simulink model "QPTest5"  (R2021a)
settings: Solver=ode45  StartTime=0.0  StopTime=20  FixedStep=Control_timestep  RelTol=1e-3  AbsTol=1e-6
undefined symbols (not defined in the file): Matlab_version, NXMotion, NXMotion_controltimestep, NXMotion_model, NXMotion_model_n, NXMotion_n, NXMotion_solution, NXMotion_solution_n, Plant_inputs_num, Plant_outputs_num
libraries: simulink x1
(part 2 of 3)

== matlab function QPTest5/MATLAB Function5 ==
  data: A input; B input; Theta0 input; XB input; P0 input; dh input; g output; q input; J input
function g = Performance_Gradient(A, B, Theta0, XB, P0, dh, q, J)
% 优化指标：
%   1) 世界坐标系 z 方向的 Directional Force Manipulability
%   2) 世界坐标系 x-y 平面的 Velocity Transmission
%   3) 世界坐标系 rx-ry 平面的 Rotational Stiffness
%
% q 顺序：
%   q(1:6)   = Stewart 六个电缸长度，单位 mm
%   q(7:13)  = 机械臂七个关节角，单位 deg

    %% -------------------------------------------------
    % 0. 固定输出尺寸与输入整理
    % --------------------------------------------------
    g = zeros(13,1);
    
    mu_const = 0;    %  w_m  10   w_s   3e-4     w_v   0.15
    
    q      = reshape(q,      13, 1);
    J      = reshape(J,       6, 13); 
    A      = reshape(A,       6, 3);
    B      = reshape(B,       6, 3);
    XB     = reshape(XB,      3, 1);
    P0     = reshape(P0,      3, 1);
    dh     = reshape(dh,      7, 4);
    Theta0 = reshape(Theta0,  7, 1);

    %% -------------------------------------------------
    % 1. 调参量
    % --------------------------------------------------
    dt = 1.0e-3;   

    % z 方向 Directional Force Manipulability 权重
    w_m = 1;  

    % rx-ry 方向 Rotational Stiffness 权重
    w_s = 0;  

    % x-y 方向 Velocity Transmission 权重
    w_v = 0; 

    % 离散加速度层缩放：
    %   q_{k+1} ≈ q_k + qdot_k*dt + 0.5*qddot_k*dt^2
    mu = mu_const * 0.5 * dt * dt;

    %% -------------------------------------------------
    % 2. 执行器力/力矩归一化矩阵 S_tau
    % --------------------------------------------------
    F_lim_cyl = 0.7 * [
        30;
        30;
        30;
        30;
        30;
        30
    ];  % N

    tau_lim_arm_Nm = 0.7 * [
        87;
        87;
        87;
        87;
        12;
        12;
        12
    ];  % Nm

    tau_lim_arm = tau_lim_arm_Nm * 1000.0;  % N*mm

    tau_lim = [
        F_lim_cyl;
        tau_lim_arm
    ];

    inv_tau = zeros(13,1);

    for i = 1:13
        inv_tau(i) = 1.0 / max(tau_lim(i), 1.0e-9);
    end

    inv_tau(13) = 0.0;

    S_tau = diag(inv_tau .* inv_tau);

    %% -------------------------------------------------
    % 2.1 关节刚度矩阵 Kq 的逆矩阵 Kq_inv
    % --------------------------------------------------
    k_cyl = 1.0e4 * [
        1;
        1;
        1;
        1;
        1;
        1
    ];  % N/mm

    k_arm_Nm_per_rad = 1.0e3 * [
        1;
        1;
        1;
        1;
        1;
        1;
        1
    ];  % Nm/rad

    k_arm = k_arm_Nm_per_rad * 1000.0;  % N*mm/rad

    k_joint = [
        k_cyl;
        k_arm
    ];

    inv_kq = zeros(13,1);

    for i = 1:13
        inv_kq(i) = 1.0 / max(k_joint(i), 1.0e-9);
    end

    inv_kq(13) = 0.0;

    Kq_inv = diag(inv_kq);

    %% -------------------------------------------------
    % 2.2 关节速度能力矩阵 S_qdot
    % --------------------------------------------------
    ldot_lim = 30.0;       % mm/s
    qdot_arm_lim = 0.50;   % rad/s

    qdot_lim = [
        ldot_lim * ones(6,1);
        qdot_arm_lim * ones(7,1)
    ];

    qdot_lim(13) = 0.0;

    S_qdot = diag(qdot_lim .* qdot_lim);

    h = zeros(13,1);

    h(1:6)  = 1.0e-2;  % Stewart 电缸，单位 mm
    h(7:12) = 1.0e-3;  % 机械臂关节，单位 deg
    h(13)   = 0.0;     % 第 7 关节固定

    qdot0 = zeros(13,1);

    grad_eta_m = zeros(13,1);
    grad_eta_s = zeros(13,1);
    grad_eta_v = zeros(13,1);

    for i = 1:12

        qp = q;
        qm = q;

        qp(i) = qp(i) + h(i);
        qm(i) = qm(i) - h(i);

        qp(13) = Theta0(7);
        qm(13) = Theta0(7);

        [Jp, ~] = System_Kinematics(A, B, XB, P0, dh, Theta0, qp, qdot0);
        [Jm, ~] = System_Kinematics(A, B, XB, P0, dh, Theta0, qm, qdot0);

        % 1) z 方向 Directional Force Manipulability
        eta_m_p = eta_dfm_z_from_J(Jp, S_tau);
        eta_m_m = eta_dfm_z_from_J(Jm, S_tau);

        % 2) rx-ry 方向 Directional Rotational Stiffness
        eta_s_p = eta_stiffness_rxy_from_J(Jp, Kq_inv);
        eta_s_m = eta_stiffness_rxy_from_J(Jm, Kq_inv);

        % 3) x-y 方向 Directional Velocity Transmission
        eta_v_p = eta_velocity_xy_from_J(Jp, S_qdot);
        eta_v_m = eta_velocity_xy_from_J(Jm, S_qdot);

        grad_eta_m(i) = (eta_m_p - eta_m_m) / (2.0 * h(i));
        grad_eta_s(i) = (eta_s_p - eta_s_m) / (2.0 * h(i));
        grad_eta_v(i) = (eta_v_p - eta_v_m) / (2.0 * h(i));
    end

    % 第 7 机械臂关节固定
    grad_eta_m(13) = 0.0;
    grad_eta_s(13) = 0.0;
    grad_eta_v(13) = 0.0;

    %% -------------------------------------------------
    % 5. 输出 QP 线性性能项
    %
    %   g = mu * (w_m * grad_eta_m
    %           + w_s * grad_eta_s
    %           + w_v * grad_eta_v)
    %
    % 其中：
    %   grad_eta_m = ∇q eta_m,z
    %   grad_eta_s = ∇q eta_s,rxy
    %   grad_eta_v = ∇q eta_v,xy
    % --------------------------------------------------
    g = mu * ( ...
          w_m * grad_eta_m ...
        + w_s * grad_eta_s ...
        + w_v * grad_eta_v );

    a=w_m * grad_eta_m';
    b=w_s * grad_eta_s';
    c=w_v * grad_eta_v';

    g(13) = 0.0;

    
end


function eta = eta_stiffness_rxy_from_J(J_ext, Kq_inv)

    J_ext  = reshape(J_ext,   6, 13);
    Kq_inv = reshape(Kq_inv, 13, 13);

    deg2rad = pi / 180.0;
    rad2deg = 180.0 / pi;


    Jk = J_ext;

    % 输出角速度/角位移单位：deg -> rad
    Jk(4:6,:) = Jk(4:6,:) * deg2rad;

    % 机械臂输入关节单位：deg -> rad
    Jk(:,7:13) = Jk(:,7:13) * rad2deg;

    % 第 7 机械臂关节固定
    Jk(:,13) = 0.0;

    Cx = Jk * Kq_inv * Jk.';
    Cx = 0.5 * (Cx + Cx.');

    scale_C = 0.0;
    for r = 1:6
        for c = 1:6
            scale_C = scale_C + Cx(r,c) * Cx(r,c);
        end
    end
    scale_C = sqrt(scale_C);

    reg = 1.0e-10 * max(scale_C, 1.0);

    Kx = (Cx + reg * eye(6)) \ eye(6);
    Kx = 0.5 * (Kx + Kx.');

    KR = Kx(4:6,4:6);
    KR = 0.5 * (KR + KR.');

    KRxy = KR(1:2,1:2);
    KRxy = 0.5 * (KRxy + KRxy.');

    eta = min_eig_sym_2x2(KRxy);

    eta = real(eta);
    eta = max(eta, 1.0e-12);

end



function eta = eta_velocity_xy_from_J(J_ext, S_qdot)


    J_ext  = reshape(J_ext,   6, 13);
    S_qdot = reshape(S_qdot, 13, 13);

    rad2deg = 180.0 / pi;


    Jv = J_ext(1:3,:);


    Jv(:,7:13) = Jv(:,7:13) * rad2deg;


    Jv(:,13) = 0.0;

    Jxy = Jv(1:2,:);

    Mv = Jxy * S_qdot * Jxy.';
    Mv = 0.5 * (Mv + Mv.');

    lambda_min = min_eig_sym_2x2(Mv);
    lambda_min = max(real(lambda_min), 1.0e-12);

    eta = sqrt(lambda_min);

end


function eta = eta_dfm_z_from_J(J_ext, S_tau)

    rad2deg = 180.0 / pi;

    ez = [
        0.0;
        0.0;
        1.0
    ];

    ez = ez / max(norm(ez), 1.0e-12);

    %% -------------------------------------------------
    % 1. 取平动 Jacobian
    % --------------------------------------------------
    Jv = J_ext(1:3,:);

    %% -------------------------------------------------
    % 2. 单位转换
    % --------------------------------------------------
    Jv(:,7:13) = Jv(:,7:13) * rad2deg;

    Jv(:,13) = 0.0;

    %% -------------------------------------------------
    % 3. z 方向 Directional Force Manipulability
    % --------------------------------------------------
    alpha = ez.' * (Jv * S_tau * Jv.') * ez;

    alpha = max(alpha, 1.0e-12);

    eta = 1.0 / sqrt(alpha);

end


function lambda_min = min_eig_sym_2x2(M)

    M = reshape(M, 2, 2);
    M = 0.5 * (M + M.');

    a = M(1,1);
    b = M(1,2);
    c = M(2,2);

    tr_half = 0.5 * (a + c);
    disc = sqrt(0.25 * (a - c) * (a - c) + b * b);

    lambda_min = tr_half - disc;

end



function [J, Jdot_qdot] = System_Kinematics (A, B, XB, P0, dh, Theta0, q, qdot)


    %% 0. 输入整理
    J = zeros(6,13);
    Jdot_qdot = zeros(6,1);

    A      = reshape(A,       6, 3);
    B      = reshape(B,       6, 3);
    XB     = reshape(XB,      3, 1);
    P0     = reshape(P0,      3, 1);
    dh     = reshape(dh,      7, 4);
    Theta0 = reshape(Theta0,  7, 1);
    q      = reshape(q,      13, 1);
    qdot   = reshape(qdot,   13, 1);

    deg2rad = pi / 180.0;
    rad2deg = 180.0 / pi;

    %% 1. 构造 qdot13，并强制第 7 机械臂关节速度为 0
    qdot13 = qdot;
    qdot13(13) = 0.0;

    %% 2. 拆分 q 与 qdot
    l_para = q(1:6);             % mm
    q_arm_deg = q(7:13);         % deg

    ldot = qdot13(1:6);          % mm/s
    qdot_arm_deg = qdot13(7:13); % deg/s

    theta7_fixed = Theta0(7);

    q_arm_deg(7) = theta7_fixed;
    qdot_arm_deg(7) = 0.0;

    q_arm_rad = q_arm_deg * deg2rad;
    qdot_arm_rad = qdot_arm_deg * deg2rad;

    %% 3. 几何参数与坐标转换
    A_G0 = A.';             % 3x6
    B_G  = B.';             % 3x6

    XB_G0 = XB(:);          % 3x1
    P0_G  = P0(:);          % 3x1

    A_P = zeros(3,6);
    for i = 1:6
        A_P(:,i) = A_G0(:,i) - P0_G;
    end

    % 机械臂基座 B 相对上平台中心 P 的安装偏置，表达在 {P}
    PpB = XB_G0 - P0_G;     % mm

    PRB = [
        -1.0,  0.0,  0.0;
         0.0, -1.0,  0.0;
         0.0,  0.0,  1.0
    ];

    % dh 中角度列 deg -> rad，长度列保持 mm
    dh_rad = dh;
    dh_rad(:,3) = dh(:,3) * deg2rad;
    dh_rad(:,4) = dh(:,4) * deg2rad;

    %% 4. Stewart 正运动学：由六个电缸长度求当前上平台位姿
    pose_guess_p = P0_G;
    pose_guess_R = eye(3);

    maxIter = 60;
    tol = 1.0e-7;

    [p_GP, R_GP] = stewart_fk_LM( ...
        A_P, B_G, l_para, ...
        pose_guess_p, pose_guess_R, ...
        maxIter, tol);

    %% 5. Stewart 速度雅可比
    [Gq, ~, ~, ~] = stewart_Gq(A_P, B_G, p_GP, R_GP);

    lambda_dls = 1.0e-3;
    A_dls  = Gq.' * Gq + lambda_dls^2 * eye(6);
    J_para = A_dls \ Gq.';

    %% 6. 机械臂 Jacobian，表达在机械臂基坐标系 {B}
    % --------------------------------------------------

    X_AEnd0_G = [-1161.7884; 0.0001; 1560.2205];

    q_arm0_deg = Theta0(:);
    q_arm0_deg(7) = Theta0(7);
    q_arm0_rad = q_arm0_deg * deg2rad;

    % 初始 MDH 末端坐标系 {F} 的位姿，p_tool_F = 0 表示先取 MDH 末端原点
    [~, T_BF0, f_F0_B, ~] = franka_jacobian_mdh_tool( ...
        q_arm0_rad, dh_rad, zeros(3,1));

    R_BF0 = T_BF0(1:3,1:3);

    % 初始时：
    %   X_AEnd0_G = XB_G0 + PRB * (f_F0_B + R_BF0*p_AEnd_F)
    %
    % 因此：
    %   p_AEnd_F = R_BF0' * ( PRB'*(X_AEnd0_G-XB_G0) - f_F0_B )
    p_AEnd_F = R_BF0.' * (PRB.' * (X_AEnd0_G - XB_G0) - f_F0_B);

    % 当前真实控制点 AEnd 的机械臂雅可比
    [J_arm_B_full, ~, f_B, Tlist] = franka_jacobian_mdh_tool( ...
        q_arm_rad, dh_rad, p_AEnd_F);
 
    % 第 7 关节固定：保留其位姿影响，但去掉速度列
    J_arm_B = J_arm_B_full;
    J_arm_B(:,7) = 0.0;

    %% 7. 组合系统总 Jacobian，内部先用 [mm/s; rad/s]
    % ^G R_B = ^G R_P * ^P R_B
    R_B = R_GP * PRB;

    % 从 P 到 AEnd 的向量，表达在 {G}
    r_PF = R_GP * PpB + R_B * f_B;

    G_PF = zeros(6,6);
    G_PF(1:3,1:3) = eye(3);
    G_PF(1:3,4:6) = -skew3(r_PF);
    G_PF(4:6,4:6) = eye(3);

    Rbar_B = zeros(6,6);
    Rbar_B(1:3,1:3) = R_B;
    Rbar_B(4:6,4:6) = R_B;

    J_stew_internal = G_PF  * J_para;
    J_arm_internal  = Rbar_B * J_arm_B;
    J_internal = [J_stew_internal, J_arm_internal];

    D_in = diag([ ...
        1; 1; 1; 1; 1; 1; ...
        deg2rad; deg2rad; deg2rad; deg2rad; deg2rad; deg2rad; deg2rad]);

    D_out = diag([1; 1; 1; rad2deg; rad2deg; rad2deg]);

    J = D_out * J_internal * D_in;
    J(:,13) = 0.0;

    %% 8. 计算 dot(J)*qdot
    % 8.1 Stewart 平台速度
    Xdot_P = J_para * ldot;
    v_P = Xdot_P(1:3);
    w_P = Xdot_P(4:6);

    % 8.2 Stewart 平台 bias 加速度
    dGq_dt  = stewart_dGq_twist(A_P, B_G, p_GP, R_GP, v_P, w_P);
    dJ_para = dls_inverse_dJ(Gq, dGq_dt, lambda_dls, A_dls, J_para);

    Xddot_P = dJ_para * ldot;
    dotv_P = Xddot_P(1:3);
    dotw_P = Xddot_P(4:6);

    % 8.3 机械臂相对 twist 和相对 bias 加速度，表达在 {B}
    Xdot_rel_B = J_arm_B * qdot_arm_rad;
    v_rel_B = Xdot_rel_B(1:3);
    w_rel_B = Xdot_rel_B(4:6);

    Xddot_rel_B = armJdotQdot_geometric_fromTlist_tool( ...
        J_arm_B, Tlist, qdot_arm_rad, f_B);

    dotv_rel_B = Xddot_rel_B(1:3);
    dotw_rel_B = Xddot_rel_B(4:6);

    % 8.4 转到世界坐标系 {G}
    v_rel_G    = R_B * v_rel_B;
    w_rel_G    = R_B * w_rel_B;
    dotv_rel_G = R_B * dotv_rel_B;
    dotw_rel_G = R_B * dotw_rel_B;

    % 8.5 末端 bias 加速度
    dotw_F_internal = dotw_P ...
                    + cross(w_P, w_rel_G) ...
                    + dotw_rel_G;

    dotv_F_internal = dotv_P ...
                    + cross(dotw_P, r_PF) ...
                    + cross(w_P, cross(w_P, r_PF)) ...
                    + 2.0 * cross(w_P, v_rel_G) ...
                    + dotv_rel_G;

    Jdot_qdot_internal = [dotv_F_internal; dotw_F_internal];
    Jdot_qdot = D_out * Jdot_qdot_internal;

    J(:,13) = 0.0;

    
    
    
    
end



%% ========================================================================
%                          Stewart FK: Levenberg-Marquardt
% ========================================================================
function [p, R] = stewart_fk_LM(A_P, B_G, l, p0, R0, maxIter, tol)
% Stewart forward kinematics by LM.
% A_P, B_G, l, p 均为 mm；旋转增量为 rad。

    p = p0(:);
    R = R0;

    lambda = 1.0e-4;
    resPrev = inf;

    for it = 1:maxIter 
        [g, Gq] = stewart_residual_and_Gq(A_P, B_G, p, R, l);
        res = norm(g);

        if res < tol
            break;
        end

        H = Gq.' * Gq + lambda * eye(6);
        delta = -(H \ (Gq.' * g));

        accepted = false;
        for trial = 1:10 
            p_new = p + delta(1:3);
            % 左扰动：delta_phi 为空间角速度/旋转增量，对应 Gq 中 -[R*A]x 项。
            R_new = so3_exp(delta(4:6)) * R;

            g_new = stewart_residual_only(A_P, B_G, p_new, R_new, l);
            res_new = norm(g_new);

            if res_new < res
                p = p_new;
                R = R_new;
                lambda = max(lambda / 5.0, 1.0e-12);
                accepted = true;
                break;
            else
                lambda = lambda * 5.0;
                H = Gq.' * Gq + lambda * eye(6);
                delta = -(H \ (Gq.' * g));
            end
        end

        if ~accepted
            break;
        end

        if abs(resPrev - res) / max(1.0, res) < 1.0e-12
            break;
        end
        resPrev = res;
    end
end

function g = stewart_residual_only(A_P, B_G, p, R, l)
    p = p(:);
    g = zeros(6,1);
    for i = 1:6
        s_i = R * A_P(:,i) + p - B_G(:,i);
        g(i) = norm(s_i) - l(i);
    end
end

function [g, Gq] = stewart_residual_and_Gq(A_P, B_G, p, R, l)
    p = p(:);
    g = zeros(6,1);
    Gq = zeros(6,6);

    rA_G = R * A_P;
    for i = 1:6
        s_i = rA_G(:,i) + p - B_G(:,i);
        L_i = norm(s_i);
        L_i_safe = max(L_i, 1.0e-12);
        u_i = s_i / L_i_safe;

        g(i) = L_i - l(i);
        Gq(i,1:3) = u_i.';
        Gq(i,4:6) = u_i.' * (-skew3(rA_G(:,i)));
    end
end

%% ========================================================================
%                          Stewart velocity Jacobian
% ========================================================================
function [Gq, u_all, rA_G_all, legVec_all] = stewart_Gq(A_P, B_G, p, R)
    p = p(:);

    Gq = zeros(6,6);
    u_all = zeros(3,6);
    rA_G_all = R * A_P;
    legVec_all = zeros(3,6);

    for i = 1:6
        s_i = rA_G_all(:,i) + p - B_G(:,i);
        L_i = norm(s_i);
        L_i_safe = max(L_i, 1.0e-12);
        u_i = s_i / L_i_safe;

        legVec_all(:,i) = s_i;
        u_all(:,i) = u_i;

        Gq(i,1:3) = u_i.';
        Gq(i,4:6) = u_i.' * (-skew3(rA_G_all(:,i)));
    end
end

%% ========================================================================
%                          Franka / 机械臂 MDH Jacobian
% ========================================================================
function [J, T_BF, f_B, Tlist] = franka_jacobian_mdh_tool(q_rad, dh_rad, p_tool_F)

    q_rad = q_rad(:);
    p_tool_F = reshape(p_tool_F, 3, 1);

    theta = q_rad + dh_rad(:,4);

    T = eye(4);
    Tlist = zeros(4,4,7);

    for i = 1:7
        a     = dh_rad(i,1);
        d     = dh_rad(i,2);
        alpha = dh_rad(i,3);
        th    = theta(i);

        Ti = mdh_T(a, d, alpha, th);
        T = T * Ti;
        Tlist(:,:,i) = T;
    end

    T_BF = T;

    R_BF = T_BF(1:3,1:3);
    p_F_B = T_BF(1:3,4);

    % AEnd 点在机械臂基坐标系 {B} 下的位置
    f_B = p_F_B + R_BF * p_tool_F;

    J = zeros(6,7);
    p_e = f_B;

    for i = 1:7
        Ti = Tlist(:,:,i);
        zi = Ti(1:3,3);
        pi = Ti(1:3,4);

        J(1:3,i) = cross(zi, p_e - pi);
        J(4:6,i) = zi;
    end
end

function T = mdh_T(a, d, alpha, theta)
% MDH: Tx(a) * Rx(alpha) * Tz(d) * Rz(theta)
% a,d: mm; alpha,theta: rad
    ca = cos(alpha);
    sa = sin(alpha);
    ct = cos(theta);
    st = sin(theta);

    T = [
        ct,    -st,     0,   a;
        st*ca, ct*ca,  -sa, -d*sa;
        st*sa, ct*sa,   ca,  d*ca;
        0,      0,      0,   1
    ];
end

%% ========================================================================
%                          dot(J_arm)*qdot_arm
% ========================================================================
function Jdotq = armJdotQdot_geometric_fromTlist_tool(J_arm_B, Tlist, qdot_rad, p_e)
% 解析计算机械臂相对项：^B(dot(J_arm)*qdot_arm)
%
% p_e:
%   AEnd 点在机械臂基坐标系 {B} 下的位置，单位 mm。
%
% 输出：
%   前3维 mm/s^2
%   后3维 rad/s^2

    qdot_rad = qdot_rad(:);
    p_e = reshape(p_e, 3, 1);

    n = 7;

    z = zeros(3,n);
    p = zeros(3,n);

    for i = 1:n
        Ti = Tlist(:,:,i);
        z(:,i) = Ti(1:3,3);
        p(:,i) = Ti(1:3,4);
    end

    v_e = J_arm_B(1:3,:) * qdot_rad;

    omega_i = zeros(3,n);
    v_i     = zeros(3,n);

    for i = 1:n
        omega_i(:,i) = z(:,1:i) * qdot_rad(1:i);

        vi = zeros(3,1);
        for k = 1:i
            vi = vi + cross(z(:,k), p(:,i) - p(:,k)) * qdot_rad(k);
        end
        v_i(:,i) = vi;
    end

    vdot_bias = zeros(3,1);
    wdot_bias = zeros(3,1);

    for i = 1:n
        zi = z(:,i);
        pi = p(:,i);

        z_dot = cross(omega_i(:,i), zi);
        wdot_bias = wdot_bias + z_dot * qdot_rad(i);

        vdot_bias = vdot_bias + ...
            ( cross(z_dot, p_e - pi) ...
            + cross(zi, v_e - v_i(:,i)) ) * qdot_rad(i);
    end

    Jdotq = [vdot_bias; wdot_bias];
end

%% ========================================================================
%                          Stewart dGq/dt
% ========================================================================
function dGq = stewart_dGq_twist(A_P, B_G, p, R, v, w)
% 计算 Stewart Gq 的时间导数。
% A_P, B_G, p: mm；v: mm/s；w: rad/s。
% Gq 定义：ldot_i = u_i^T v_P + u_i^T(-[rAi]x) w_P。

    p = p(:);
    v = v(:);
    w = w(:);

    dGq = zeros(6,6);
    rA = R * A_P;

    for i = 1:6
        rAi = rA(:,i);
        s_i = rAi + p - B_G(:,i);

        L_i = norm(s_i);
        L_i_safe = max(L_i, 1.0e-12);
        u_i = s_i / L_i_safe;

        ds = v + cross(w, rAi);
        dL = u_i.' * ds;
        du = (ds - u_i * dL) / L_i_safe;

        drAi = cross(w, rAi);

        dGq(i,1:3) = du.';
        dGq(i,4:6) = du.' * (-skew3(rAi)) ...
                   + u_i.' * (-skew3(drAi));
    end
end

%% ========================================================================
%                          DLS inverse derivative
% ========================================================================
function dJ = dls_inverse_dJ(G, dG, lambda_dls, A, J)
% J = inv(G^T G + lambda^2 I)*G^T 的时间导数。
% dJ = A^{-1} dG^T - A^{-1}(dG^T G + G^T dG)J

    if nargin < 4
        A = G.' * G + lambda_dls^2 * eye(size(G,2));
    end
    if nargin < 5
        J = A \ G.';
    end

    dA = dG.' * G + G.' * dG;
    dJ = (A \ dG.') - (A \ (dA * J));
end

%% ========================================================================
%                          Basic SO(3) functions
% ========================================================================
function S = skew3(v)
    v = v(:);
    S = [
          0,   -v(3),  v(2);
        v(3),    0,  -v(1);
       -v(2),  v(1),    0
    ];
end

function R = so3_exp(w)
    w = w(:);
    th = norm(w);

    if th < 1.0e-12
        R = eye(3) + skew3(w);
        return;
    end

    k = w / th;
    K = skew3(k);
    R = eye(3) + sin(th) * K + (1.0 - cos(th)) * (K * K);
end

== matlab function QPTest5/MATLAB Function6 ==
  data: qdot_cmd_output output; t input; A input; B input; Theta0 input; qddot_cmd input; q input; qdot_in input
function qdot_cmd_output  = Command_Integrator( ...
     t, A, B, Theta0, qddot_cmd, q, qdot_in)


    %% -------------------------------------------------
    % 0. 固定输出尺寸与输入整理
    % --------------------------------------------------
    qdot_cmd_output = zeros(12,1);

    qddot_cmd = reshape(qddot_cmd, 13, 1);
    q          = reshape(q,          13, 1);
    qdot_in    = reshape(qdot_in,    13, 1);
    A          = reshape(A,           6, 3);
    B          = reshape(B,           6, 3);

    %% -------------------------------------------------
    % 0.1 启动保护
    % --------------------------------------------------
    t_start = 2.0e-3;   % s

    if t < t_start
        qdot_cmd_output(:) = 0.0;
        return;
    end

    %% -------------------------------------------------
    % 1. Theta0 处理
    % --------------------------------------------------
    Theta0_vec = Theta0(:);
    nTheta0 = numel(Theta0_vec);

    if nTheta0 >= 7
        theta7_fixed = Theta0_vec(7);
    else
        theta7_fixed = Theta0_vec(1);
    end

    %% -------------------------------------------------
    % 2. 内部 13 维 qdot
    % --------------------------------------------------
    qdot = qdot_in;

    %% -------------------------------------------------
    % 3. 控制周期
    % --------------------------------------------------
    dt = 1.0000e-03;     % s

    %% -------------------------------------------------
    % 4. 由 A、B 计算 Stewart 初始长度 L0
    % --------------------------------------------------
    dAB = A - B;
    L0 = zeros(6,1);

    for i = 1:6
        L0(i) = sqrt(dAB(i,1)*dAB(i,1) + ...
                     dAB(i,2)*dAB(i,2) + ...
                     dAB(i,3)*dAB(i,3));
    end

    %% -------------------------------------------------
    % 5. 第 7 关节固定处理
    % --------------------------------------------------
    q(13)         = theta7_fixed;
    qdot(13)      = 0.0;
    qddot_cmd(13) = 0.0;

    %% -------------------------------------------------
    % 6. 基本限幅参数
    % --------------------------------------------------
    rad2deg = 180.0 / pi;

    q_min = zeros(13,1);
    q_max = zeros(13,1);

    stroke_half = 100.0;     % mm

    q_min(1:6) = L0 - stroke_half;
    q_max(1:6) = L0 + stroke_half;

    theta_min_rad = [
        -2.8973;
        -1.7628;
        -2.8973;
        -3.0718;
        -2.8973;
        -0.0175;
        -2.8973
    ];

    theta_max_rad = [
         2.8973;
         1.7628;
         2.8973;
        -0.0698;
         2.8973;
         3.7525;
         2.8973
    ];

    theta_min = theta_min_rad * rad2deg;
    theta_max = theta_max_rad * rad2deg;

    q_min(7:13) = theta_min;
    q_max(7:13) = theta_max;

    q_min(13) = theta7_fixed;
    q_max(13) = theta7_fixed;

    qdot_min = zeros(13,1);
    qdot_max = zeros(13,1);

    ldot_max = 30.0;                % mm/s
    thetadot_max = 0.50 * rad2deg;  % deg/s

    qdot_min(1:6)  = -ldot_max;
    qdot_max(1:6)  =  ldot_max;

    qdot_min(7:12) = -thetadot_max;
    qdot_max(7:12) =  thetadot_max;

    qdot_min(13) = 0.0;
    qdot_max(13) = 0.0;

    qddot_min = zeros(13,1);
    qddot_max = zeros(13,1);

    lddot_max = 200.0;               % mm/s^2
    thetaddot_max = 1.00 * rad2deg;  % deg/s^2

    qddot_min(1:6)  = -lddot_max;
    qddot_max(1:6)  =  lddot_max;

    qddot_min(7:12) = -thetaddot_max;
    qddot_max(7:12) =  thetaddot_max;

    qddot_min(13) = 0.0;
    qddot_max(13) = 0.0;

    %% -------------------------------------------------
    % 7. 对 qddot_cmd 做安全限幅
    % --------------------------------------------------
    qddot_safe = sat_vec13(qddot_cmd, qddot_min, qddot_max);

    %% -------------------------------------------------
    % 8. 加速度积分为速度指令
    % --------------------------------------------------
    qdot_des = qdot + qddot_safe * dt;
    
    %% -------------------------------------------------
    % 9. 速度限幅
    % --------------------------------------------------
    qdot_des = sat_vec13(qdot_des, qdot_min, qdot_max);

    %% -------------------------------------------------
    % 10. 位置保护
    % --------------------------------------------------
    qdot_cmd = zeros(13,1);

    for i = 1:13

        lb_pos = (q_min(i) - q(i)) / dt;
        ub_pos = (q_max(i) - q(i)) / dt;

        lb = max(qdot_min(i), lb_pos);
        ub = min(qdot_max(i), ub_pos);

        if lb <= ub
            qdot_cmd(i) = sat_scalar(qdot_des(i), lb, ub);
        else
            if q(i) < q_min(i)
                qdot_cmd(i) = qdot_max(i);
            elseif q(i) > q_max(i)
                qdot_cmd(i) = qdot_min(i);
            else
                qdot_cmd(i) = 0.0;
            end
        end
    end

    
    %% -------------------------------------------------
    % 11. 第 7 关节固定，并输出 12 个有效速度
    % --------------------------------------------------
    qdot_cmd(13) = 0.0;

    qdot_cmd_output(1:12) = qdot_cmd(1:12);

end

%% ========================================================================
%                         helper: 13x1 vector saturation
% ========================================================================

function y = sat_vec13(x, lb, ub)
    y = zeros(13,1);

    for i = 1:13
        y(i) = sat_scalar(x(i), lb(i), ub(i));
    end
end

%% ========================================================================
%                         helper: scalar saturation
% ========================================================================

function y = sat_scalar(x, lb, ub)

    if ~isfinite(x)
        x = 0.0;
    end

    if ~isfinite(lb)
        lb = -realmax;
    end

    if ~isfinite(ub)
        ub = realmax;
    end

    y = x;

    if y < lb
        y = lb;
    end

    if y > ub
        y = ub;
    end
end

== matlab function QPTest5/MATLAB Function7 ==
  data: t input; Xddot_des input; A input; B input; Theta0 input; g input; q input; qdot_in input; J input; Jdot_qdot input; qddot_cmd output; eta_m_z output; eta_s_rxy output; eta_v_xy output
function [qddot_cmd, eta_m_z, eta_s_rxy, eta_v_xy] = QP_Builder_Solver( ...
     t, Xddot_des, A, B, Theta0, g, q, qdot_in, J, Jdot_qdot)

% 当前外部单位：
%   长度：mm
%   角度：deg
%
% 输入：
%   t             当前时间，单位 s
%   J             6x13 系统雅可比矩阵
%   Jdot_qdot     6x1  dot(J)*dot(q)
%   Xddot_des     6x1  期望末端笛卡尔加速度
%   g             13x1 性能梯度线性项
%   q             13x1 当前系统广义坐标
%   qdot_in       13x1 当前系统广义速度反馈
%
% 输出：
%   qddot_cmd     13x1 关节加速度命令
%   eta_m_z       z 方向 Directional Force Manipulability
%   eta_s_rxy     rx-ry 方向 Rotational Stiffness
%   eta_v_xy      x-y 方向 Velocity Transmission
%
% QP 目标：
%   min  (J*qddot + Jdot_qdot - Xddot_des)' * Wx *
%        (J*qddot + Jdot_qdot - Xddot_des)
%        + qddot' * Wq * qddot
%        - g' * qddot


    %% -------------------------------------------------
    % 0. 固定输出尺寸与输入整理
    % --------------------------------------------------
    qddot_cmd = zeros(13,1);

    J          = reshape(J,          6, 13);
    Jdot_qdot = reshape(Jdot_qdot,   6, 1);
    Xddot_des = reshape(Xddot_des,   6, 1);
    g          = reshape(g,         13, 1);
    q          = reshape(q,         13, 1);
    qdot_in    = reshape(qdot_in,   13, 1);
    A          = reshape(A,          6, 3);
    B          = reshape(B,          6, 3);

    eta_m_z   = 0.0;
    eta_s_rxy = 0.0;
    eta_v_xy  = 0.0;

    %% -------------------------------------------------
    % 0.1 启动保护
    % --------------------------------------------------
    t_start = 2.0e-3;   % s

    if t < t_start
        qddot_cmd(:) = 0.0;
        return;
    end

    %% -------------------------------------------------
    % 0.2 NaN / Inf 保护
    % --------------------------------------------------
    if has_bad_mat_6x13(J) || has_bad_vec6(Jdot_qdot) || has_bad_vec6(Xddot_des)
        qddot_cmd(:) = 0.0;
        return;
    end

    % 兼容 Theta0 为 7x1 或 1x1 的情况
    Theta0_vec = Theta0(:);
    if numel(Theta0_vec) >= 7
        theta7_fixed = Theta0_vec(7);
    else
        theta7_fixed = Theta0_vec(1);
    end

    % 构造内部 13 维 qdot
    qdot = qdot_in;

    q(13)     = theta7_fixed;
    qdot(13)  = 0.0;
    J(:,13)   = 0.0;
    g(13)     = 0.0;


    %% -------------------------------------------------
    % 1. 控制周期
    % --------------------------------------------------
    dt = 1.0000e-03;     % s

    %% -------------------------------------------------
    % 2. 单位转换矩阵
    % --------------------------------------------------
    mm_to_m = 1.0e-3;
    m_to_mm = 1.0e3;

    deg2rad = pi / 180.0;
    rad2deg = 180.0 / pi;

    Dq = diag([
        mm_to_m;
        mm_to_m;
        mm_to_m;
        mm_to_m;
        mm_to_m;
        mm_to_m;
        deg2rad;
        deg2rad;
        deg2rad;
        deg2rad;
        deg2rad;
        deg2rad;
        deg2rad
    ]);

    Dq_inv = diag([
        m_to_mm;
        m_to_mm;
        m_to_mm;
        m_to_mm;
        m_to_mm;
        m_to_mm;
        rad2deg;
        rad2deg;
        rad2deg;
        rad2deg;
        rad2deg;
        rad2deg;
        rad2deg
    ]);

    Dx = diag([
        mm_to_m;
        mm_to_m;
        mm_to_m;
        deg2rad;
        deg2rad;
        deg2rad
    ]);

    %% -------------------------------------------------
    % 3. 转换到内部 m/rad 单位
    % --------------------------------------------------
    J_phy = Dx * J * Dq_inv;

    Jdot_qdot_phy = Dx * Jdot_qdot;
    Xddot_des_phy = Dx * Xddot_des;

    g_phy = Dq_inv.' * g;

    J_phy(:,13) = 0.0;
    g_phy(13) = 0.0;

    %% -------------------------------------------------
    % 3.1 当前性能指标计算
    % --------------------------------------------------
    [S_tau_metric, Kq_inv_metric, S_qdot_metric] = build_metric_mats_qp();

    eta_m_z   = eta_dfm_z_from_J_qp(J, S_tau_metric);
    eta_s_rxy = eta_stiffness_rxy_from_J_qp(J, Kq_inv_metric);
    eta_v_xy  = eta_velocity_xy_from_J_qp(J, S_qdot_metric);

    if ~isfinite(eta_m_z)
        eta_m_z = 0.0;
    end

    if ~isfinite(eta_s_rxy)
        eta_s_rxy = 0.0;
    end

    if ~isfinite(eta_v_xy)
        eta_v_xy = 0.0;
    end

    %% -------------------------------------------------
    % 3.2 固定短时间窗口启用 g，并限制 g 的关节分配
    % --------------------------------------------------

    g_window_start = 0.020;    % s
    g_window_end   = 10;       % s
    g_ramp_time    = 0.100;    % s

    gamma_g = 0.0;

    window_len = g_window_end - g_window_start;

    if window_len <= 1.0e-9
        gamma_g = 0.0;
    else
        if g_ramp_time > 0.5 * window_len
            g_ramp = 0.5 * window_len;
        else
            g_ramp = g_ramp_time;
        end

        if g_ramp <= 1.0e-9
            if t >= g_window_start && t <= g_window_end
                gamma_g = 1.0;
            else
                gamma_g = 0.0;
            end
        else
            if t < g_window_start
                gamma_g = 0.0;

            elseif t < g_window_start + g_ramp
                gamma_g = (t - g_window_start) / g_ramp;

            elseif t <= g_window_end - g_ramp
                gamma_g = 1.0;

            elseif t < g_window_end
                gamma_g = (g_window_end - t) / g_ramp;

            else
                gamma_g = 0.0;
            end
        end
    end

    if gamma_g < 0.0
        gamma_g = 0.0;
    end

    if gamma_g > 1.0
        gamma_g = 1.0;
    end


    g_scale = zeros(13,1);
    
    g_scale(1:6) = 0.10;
    g_scale(7:12) = 0.10;

    g_phy = gamma_g * (g_scale .* g_phy);

    g_phy(13) = 0.0;

    %% -------------------------------------------------
    % 4. QP 权重矩阵
    % --------------------------------------------------
    Wx = diag([
        1.0;
        1.0;
        3.0;
        0.2;
        0.2;
        0.2
    ]);

    Wq_diag = zeros(13,1);
  
    Wq_diag(1:6)   = 1.0e-3;   % Stewart 电缸   1.0e-3
    Wq_diag(7:12)  = 1.0e-4;   % 机械臂前 6 关节  1.0e-4
    Wq_diag(13)    = 1.0;     

    Wq = diag(Wq_diag);

    %% -------------------------------------------------
    % 5. 构造 QP 标准形式
    % --------------------------------------------------
    b_phy = Xddot_des_phy - Jdot_qdot_phy;

    H = 2.0 * (J_phy.' * Wx * J_phy + Wq);
    f = -2.0 * (J_phy.' * Wx * b_phy) - g_phy;

    H = 0.5 * (H + H.') + 1.0e-9 * eye(13);

    if has_bad_mat_13x13(H) || has_bad_vec13(f)
        qddot_cmd(:) = 0.0;
        return;
    end

    %% -------------------------------------------------
    % 6. 关节位置、速度、加速度限制
    % --------------------------------------------------
    dAB = A - B;
    L0 = sqrt(sum(dAB.^2, 2));       % 6x1, mm

    q_min = zeros(13,1);
    q_max = zeros(13,1);

    stroke = 800.0;     % mm

    q_min(1:6) = L0 - stroke;
    q_max(1:6) = L0 + stroke;

    theta_min_rad = [
        -2.8973;
        -1.7628;
        -2.8973;
        -3.0718;
        -2.8973;
        -0.0175;
        -2.8973
    ];

    theta_max_rad = [
         2.8973;
         1.7628;
         2.8973;
        -0.0698;
         2.8973;
         3.7525;
         2.8973
    ];

    theta_min = theta_min_rad * rad2deg;
    theta_max = theta_max_rad * rad2deg;

    q_min(7:13) = theta_min;
    q_max(7:13) = theta_max;

    q_min(13) = theta7_fixed;
    q_max(13) = theta7_fixed;

    qdot_min = zeros(13,1);
    qdot_max = zeros(13,1);

    ldot_max = 30.0;                  % mm/s
    thetadot_max = 0.50 * rad2deg;    % deg/s

    qdot_min(1:6)  = -ldot_max;
    qdot_max(1:6)  =  ldot_max;

    qdot_min(7:12) = -thetadot_max;
    qdot_max(7:12) =  thetadot_max;

    qdot_min(13) = 0.0;
    qdot_max(13) = 0.0;

    qddot_min = zeros(13,1);
    qddot_max = zeros(13,1);

    lddot_max = 200.0;                % mm/s^2
    thetaddot_max = 1.00 * rad2deg;   % deg/s^2

    qddot_min(1:6)  = -lddot_max;
    qddot_max(1:6)  =  lddot_max;

    qddot_min(7:12) = -thetaddot_max;
    qddot_max(7:12) =  thetaddot_max;

    qddot_min(13) = 0.0;
    qddot_max(13) = 0.0;

    %% -------------------------------------------------
    % 7. 转换为 qddot 上下界
    % --------------------------------------------------
    lb_ext = zeros(13,1);
    ub_ext = zeros(13,1);

    for i = 1:13
        lb_acc = qddot_min(i);
        ub_acc = qddot_max(i);

        lb_vel = (qdot_min(i) - qdot(i)) / dt;
        ub_vel = (qdot_max(i) - qdot(i)) / dt;

        lb_pos = 2.0 * (q_min(i) - q(i) - qdot(i)*dt) / (dt*dt);
        ub_pos = 2.0 * (q_max(i) - q(i) - qdot(i)*dt) / (dt*dt);

        lb_ext(i) = max(lb_acc, max(lb_vel, lb_pos));
        ub_ext(i) = min(ub_acc, min(ub_vel, ub_pos));
    end

    lb_ext(13) = 0.0;
    ub_ext(13) = 0.0;

    % 若当前状态已经越界导致 lb > ub，使用制动加速度保底
    for i = 1:13
        if lb_ext(i) > ub_ext(i)
            brake = -qdot(i) / dt;

            if brake < qddot_min(i)
                brake = qddot_min(i);
            end

            if brake > qddot_max(i)
                brake = qddot_max(i);
            end

            lb_ext(i) = brake;
            ub_ext(i) = brake;
        end
    end

    lb_ext(13) = 0.0;
    ub_ext(13) = 0.0;

    %% -------------------------------------------------
    % 8. 转换为内部单位
    % --------------------------------------------------
    lb_phy = Dq * lb_ext;
    ub_phy = Dq * ub_ext;

    %% -------------------------------------------------
    % 9. 求解带上下界约束的 QP
    % --------------------------------------------------
    qddot_phy = box_qp_projected_gradient_13(H, f, lb_phy, ub_phy);

    if has_bad_vec13(qddot_phy)
        qddot_cmd(:) = 0.0;
        return;
    end

    qddot_cmd = Dq_inv * qddot_phy;

    qddot_cmd = project_box_13(qddot_cmd, lb_ext, ub_ext);

    qddot_cmd(13) = 0.0;

end


%% ========================================================================
%                    Bound-constrained QP solver
% ========================================================================

function x = box_qp_projected_gradient_13(H, f, lb, ub)

    x = zeros(13,1);

    x0 = -(H \ f);

    if has_bad_vec13(x0)
        x0 = zeros(13,1);
    end

    x = project_box_13(x0, lb, ub);

    L = 0.0;
    for i = 1:13
        for j = 1:13
            L = L + H(i,j) * H(i,j);
        end
    end

    L = sqrt(L);

    if L < 1.0e-12
        L = 1.0;
    end

    alpha = 1.0 / L;

    maxIter = 100;
    tol = 1.0e-8;

    for k = 1:maxIter
        grad = H * x + f;

        x_new = project_box_13(x - alpha * grad, lb, ub);

        dx = x_new - x;

        if sqrt(sum(dx.^2)) <= tol * (1.0 + sqrt(sum(x.^2)))
            x = x_new;
            break;
        end

        x = x_new;
    end

end

%% ========================================================================
%                    Projection onto box constraints
% ========================================================================

function y = project_box_13(x, lb, ub)

    y = zeros(13,1);

    for i = 1:13
        yi = x(i);

        if yi < lb(i)
            yi = lb(i);
        end

        if yi > ub(i)
            yi = ub(i);
        end

        y(i) = yi;
    end

end

%% ========================================================================
%                    Performance metric matrices
% ========================================================================

function [S_tau, Kq_inv, S_qdot] = build_metric_mats_qp()

    %% -------------------------------------------------
    % 1. 执行器力/力矩归一化矩阵 S_tau
    % --------------------------------------------------
    F_lim_cyl = 0.7 * [
        30;
        30;
        30;
        30;
        30;
        30
    ];  % N

    tau_lim_arm_Nm = 0.7 * [
        87;
        87;
        87;
        87;
        12;
        12;
        12
    ];  % Nm

    tau_lim_arm = tau_lim_arm_Nm * 1000.0;  % N*mm

    tau_lim = [
        F_lim_cyl;
        tau_lim_arm
    ];

    inv_tau = zeros(13,1);

    for i = 1:13
        inv_tau(i) = 1.0 / max(tau_lim(i), 1.0e-9);
    end

    % 第 7 机械臂关节固定
    inv_tau(13) = 0.0;

    S_tau = diag(inv_tau .* inv_tau);

    %% -------------------------------------------------
    % 2. 关节刚度矩阵 Kq 的逆矩阵 Kq_inv
    % --------------------------------------------------
    k_cyl = 1.0e4 * [
        1;
        1;
        1;
        1;
        1;
        1
    ];  % N/mm

    k_arm_Nm_per_rad = 1.0e3 * [
        1;
        1;
        1;
        1;
        1;
        1;
        1
    ];  % Nm/rad

    k_arm = k_arm_Nm_per_rad * 1000.0;  % N*mm/rad

    k_joint = [
        k_cyl;
        k_arm
    ];

    inv_kq = zeros(13,1);

    for i = 1:13
        inv_kq(i) = 1.0 / max(k_joint(i), 1.0e-9);
    end

    % 第 7 机械臂关节固定
    inv_kq(13) = 0.0;

    Kq_inv = diag(inv_kq);

    %% -------------------------------------------------
    % 3. 关节速度能力矩阵 S_qdot
    % --------------------------------------------------
    ldot_lim = 30.0;       % mm/s
    qdot_arm_lim = 0.50;   % rad/s

    qdot_lim = [
        ldot_lim * ones(6,1);
        qdot_arm_lim * ones(7,1)
    ];

    % 第 7 机械臂关节固定
    qdot_lim(13) = 0.0;

    S_qdot = diag(qdot_lim .* qdot_lim);

end

%% ========================================================================
%                    z-direction force manipulability
% ========================================================================

function eta = eta_dfm_z_from_J_qp(J_ext, S_tau)

    J_ext = reshape(J_ext, 6, 13);
    S_tau = reshape(S_tau, 13, 13);

    rad2deg = 180.0 / pi;

    ez = [
        0.0;
        0.0;
        1.0
    ];

    ez = ez / max(norm(ez), 1.0e-12);

    Jv = J_ext(1:3,:);

    % Arm 列由 mm/deg 转为 mm/rad
    Jv(:,7:13) = Jv(:,7:13) * rad2deg;

    % 第 7 机械臂关节固定
    Jv(:,13) = 0.0;

    alpha = ez.' * (Jv * S_tau * Jv.') * ez;
    alpha = max(alpha, 1.0e-12);

    eta = 1.0 / sqrt(alpha);
    eta = real(eta);
    eta = max(eta, 1.0e-12);

end

%% ========================================================================
%                    rx-ry rotational stiffness
% ========================================================================

function eta = eta_stiffness_rxy_from_J_qp(J_ext, Kq_inv)

    J_ext  = reshape(J_ext,   6, 13);
    Kq_inv = reshape(Kq_inv, 13, 13);

    deg2rad = pi / 180.0;
    rad2deg = 180.0 / pi;

    Jk = J_ext;

    % 输出角速度/角位移单位：deg -> rad
    Jk(4:6,:) = Jk(4:6,:) * deg2rad;

    % 机械臂输入关节单位：deg -> rad
    Jk(:,7:13) = Jk(:,7:13) * rad2deg;

    % 第 7 机械臂关节固定
    Jk(:,13) = 0.0;

    Cx = Jk * Kq_inv * Jk.';
    Cx = 0.5 * (Cx + Cx.');

    scale_C = 0.0;
    for r = 1:6
        for c = 1:6
            scale_C = scale_C + Cx(r,c) * Cx(r,c);
        end
    end
    scale_C = sqrt(scale_C);

    reg = 1.0e-10 * max(scale_C, 1.0);

    Kx = (Cx + reg * eye(6)) \ eye(6);
    Kx = 0.5 * (Kx + Kx.');

    KR = Kx(4:6,4:6);
    KR = 0.5 * (KR + KR.');

    KRxy = KR(1:2,1:2);
    KRxy = 0.5 * (KRxy + KRxy.');

    eta = min_eig_sym_2x2_qp(KRxy);

    eta = real(eta);
    eta = max(eta, 1.0e-12);

end

%% ========================================================================
%                    x-y velocity transmission
% ========================================================================

function eta = eta_velocity_xy_from_J_qp(J_ext, S_qdot)

    J_ext  = reshape(J_ext,   6, 13);
    S_qdot = reshape(S_qdot, 13, 13);

    rad2deg = 180.0 / pi;

    Jv = J_ext(1:3,:);

    % Arm 列由 mm/deg 转为 mm/rad
    Jv(:,7:13) = Jv(:,7:13) * rad2deg;

    % 第 7 机械臂关节固定
    Jv(:,13) = 0.0;

    Jxy = Jv(1:2,:);

    Mv = Jxy * S_qdot * Jxy.';
    Mv = 0.5 * (Mv + Mv.');

    lambda_min = min_eig_sym_2x2_qp(Mv);
    lambda_min = max(real(lambda_min), 1.0e-12);

    eta = sqrt(lambda_min);
    eta = real(eta);
    eta = max(eta, 1.0e-12);

end

%% ========================================================================
%                    2x2 symmetric min eigenvalue
% ========================================================================

function lambda_min = min_eig_sym_2x2_qp(M)

    M = reshape(M, 2, 2);
    M = 0.5 * (M + M.');

    a = M(1,1);
    b = M(1,2);
    c = M(2,2);

    tr_half = 0.5 * (a + c);
    disc = sqrt(0.25 * (a - c) * (a - c) + b * b);

    lambda_min = tr_half - disc;

end

%% ========================================================================
%                    finite checks
% ========================================================================

function bad = has_bad_vec6(x)
    bad = false;
    for i = 1:6
        if ~isfinite(x(i))
            bad = true;
            return;
        end
    end
end

function bad = has_bad_vec13(x)
    bad = false;
    for i = 1:13
        if ~isfinite(x(i))
            bad = true;
            return;
        end
    end
end

function bad = has_bad_mat_6x13(A)
    bad = false;
    for i = 1:6
        for j = 1:13
            if ~isfinite(A(i,j))
                bad = true;
                return;
            end
        end
    end
end

function bad = has_bad_mat_13x13(A)
bad = false;
for i = 1:13
    for j = 1:13
        if ~isfinite(A(i,j))
            bad = true;
            return;
        end
    end
end
end
